simulink model "Project3"  (R2014a)
settings: Solver=ode45  StartTime=0.0  StopTime=Sim_Time  MaxStep=0.01  RelTol=1e-3
values from neighbouring files (symbols this model uses):
  b = 3    [Project3_Run.m]
  F = 1    [Project3_Run.m]
  k = 20    [Project3_Run.m]
  M = 1    [Project3_Run.m]
settings Model: Creator=dzr3qn  LastModifiedBy=DZR3QN

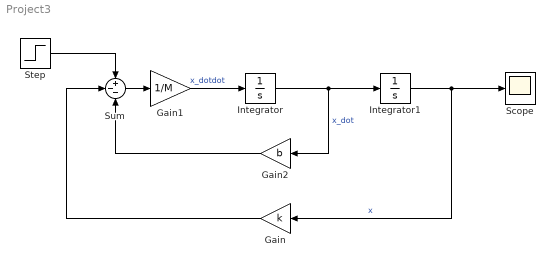
== system Project3 ==
  Gain : Gain  Gain=k
  Gain1 : Gain  Gain=1/M
  Gain2 : Gain  Gain=b
  Integrator : Integrator
  Integrator1 : Integrator
  Scope : Scope
  Step : Step  Time=0.1  After=F  SampleTime=0
  Sum : Sum  Inputs=+--
  wires:
  Integrator/1 -> Gain2/1, Integrator1/1  "x_dot"
  Integrator1/1 -> Scope/1, Gain/1  "x"
  Sum/1 -> Gain1/1
  Gain1/1 -> Integrator/1  "x_dotdot"
  Gain2/1 -> Sum/3
  Gain/1 -> Sum/2
  Step/1 -> Sum/1
